simulink model "TruckBenchmark"  (R2023a)
settings: Solver=FixedStepAuto  StartTime=0.0  StopTime=sim_time  FixedStep=control.Ts  MaxStep=1  RelTol=1e-3  EnableMultiTasking=on
StartFcn:
  | tic
StopFcn:
  | simt=toc;
  | fprintf('Simulation time %.3f s\n',simt)
  | TruckBenchmark_Evaluation
values from neighbouring files (symbols this model uses):
  attack_duration = input('Enter the duration of each attack: ')    [RunMe.m]
  attack_freq = input('Enter the desired frequency of attack: ')    [RunMe.m]
  attack_time = input('Enter the time for attack: ')    [RunMe.m]
  attack_type = input('Select the type of Attack (1= Fuzzy, 2=spoofing, 3=Plateau, 4=Replay Attack, 5 = GAttack, 6= C-GAttack, 7= No Attack, 8 = Denial of Service):')    [RunMe.m]
  can_sample_time = 0.001    [runSim.m]
  clutch_pos = TruckBenchmark_Result.find('clutch_pos').Values    [TruckBenchmark_Evaluation.m]
  control =     [TruckBenchmark_Control.mat]
  cruise_profile = input('Select Cruise Profile (Step decrease = 1, Constant 80kph = 2): ')    [RunMe.m]
  curr_gear = TruckBenchmark_Result.find('curr_gear').Values    [TruckBenchmark_Evaluation.m]
  DoS = 0    [RunMe.m]
  gattack_data = interp1(original_time, data, desired_time, 'linear')    [RunMe.m]
  gattack_time = desired_time    [RunMe.m]
  k_slope = TruckBenchmark_Result.find('k_slope').Values    [TruckBenchmark_Evaluation.m]
  lambda = TruckBenchmark_Result.find('lambda').Values    [TruckBenchmark_Evaluation.m]
  model =     [TruckBenchmark_Data.mat]
  n_engine = TruckBenchmark_Result.find('n_engine').Values    [TruckBenchmark_Evaluation.m]
  road = scenario.road    [runSim.m]
  scenario =     [Sodertalje_Norrkoping_Scenario.mat]
  sim_time = input('Enter the total simulation time: ')    [RunMe.m]
  spoofed_value = input('Set the spoofing value:')    [RunMe.m]
  ts = struct('orig_30kph', ts_orig_30kph, 'gen_30kph', ts_gen_30kph, 'orig_40kph', ts_orig_40kph, 'gen_40kph', ts_gen_40kph, 'orig_50kph', ts_orig_50kph, 'gen_50kph', ts_gen_50kph, 'orig_60kph', ts_orig_60kph, 'gen_60kph', ts_gen_60kph,'orig_70kph', ts_orig_70kph, 'gen_70kph', ts_gen_70kph, 'orig_80kph', ts_orig_80kph, 'gen_80kph', ts_gen_80kph, 'orig_90kph', ts_orig_90kph, 'gen_90kph', ts_gen_90kph)    [data_to_mat.m]
  v_vehicle = 0    [RunMe.m]    (also in TruckBenchmark_Evaluation.m = TruckBenchmark_Result.find('v_vehicle').Values)
undefined symbols (not defined in the file or in its folder): canChannel, CCVS, DiscIntNeverNeededParam, dm_airInlet, EGF1, ESSI, ETC2, gcbh, IMT1, n_t, p_inletManifold, r_egr, VD, VDHR, x_distance
libraries: j1939protocollib x25, simulink x5, canlib x2, j1939tllib x2, canmsglib x1, vntj1939tllib x1, slpidlib x1
(part 3 of 4)

== system TruckBenchmark/Controller/CAN TX//RX/J1939 CAN Transport Layer3 ==
  CAN Configuration : S-Function  LoadFcn=set_param(gcb, 'BlockHandle', num2str(gcbh));  FunctionName=svntcanconfig  Parameters=BlockHandle, Device, ObjConstructor, BusSpeed, EnableBitParameters, SJW, TSEG1, TSEG2, NSamples, AckMode  SFunctionDeploymentMode=off  EnableBusSupport=off  mask(CAN Configuration){BlockHandle=865.0001, Device=MathWorks Virtual 1 (Channel 2), ObjConstructor=canChannel('MathWorks', 'Virtual 1', 2), BusSpeed=250000, EnableBitParameters=off, SJW=1, TSEG1=4, TSEG2=3, NSamples=1, AckMode=Normal}
      mask prompts: BlockHandle "Block handle"; Device "Device Name"; ObjConstructor "Object constructor"; BusSpeed "Bus speed:"; EnableBitParameters "Set bit parameters manually"; SJW "Synchronization jump width (SJW):"; TSEG1 "Time segment 1 (TSEG1)"; TSEG2 "Time segment 2 (TSEG2)"; NSamples "Number of samples:"; AckMode "Acknowledge mode:"
      mask help: Configure the properties for the specified CAN device.
      mask Help: eval('helpview(fullfile(docroot, ''toolbox'', ''vnt'', ''vnt.map''), ''vnt_canconfig_block'')');
      mask TypeOptions AckMode: Normal | Silent
  CAN Receive : S-Function  LoadFcn=set_param(gcb, 'BlockHandle', num2str(gcbh));  FunctionName=svntcanreceive  Parameters=BlockHandle, Device, ObjConstructor, EnableStandardIDsFilter, StandardIDs, EnableExtendedIDsFilter, ExtendedIDs, SampleTime, MsgsPerTimestep, StdIDsCombo, ExtIDsCombo, InternalFilterUpdateStatus, BusOutput  SFunctionDeploymentMode=off  EnableBusSupport=off  mask(CAN Receive){BlockHandle=866.0004, Device=MathWorks Virtual 1 (Channel 2), ObjConstructor=canChannel('MathWorks', 'Virtual 1', 2), EnableStandardIDsFilter=off, StandardIDs=0, EnableExtendedIDsFilter=off, ExtendedIDs=0, SampleTime=can_sample_time, MsgsPerTimestep=all, StdIDsCombo=Allow all, ExtIDsCombo=Allow all, InternalFilterUpdateStatus=on, BusOutput=off}
      mask prompts: BlockHandle "Block handle"; Device "Device Name"; ObjConstructor "Object constructor"; EnableStandardIDsFilter "Filter for accepted Standard ID range"; StandardIDs "Standard IDs"; EnableExtendedIDsFilter "Filter for accepted Extended ID range"; ExtendedIDs "Extended IDs"; SampleTime "Sample time:"; MsgsPerTimestep "Messages per timestep"; StdIDsCombo "Standard IDs Combo"; ExtIDsCombo "Extended IDs Combo"; InternalFilterUpdateStatus "Internal Filter update"; BusOutput "Output as bus"
      mask help: Receive CAN Messages using the specified CAN device.
      mask Help: eval('helpview(fullfile(docroot, ''toolbox'', ''vnt'', ''vnt.map''), ''vnt_canrec_block'')');
      mask TypeOptions MsgsPerTimestep: 1 | all
      mask TypeOptions StdIDsCombo: Allow all | Allow only | Block only
      mask TypeOptions ExtIDsCombo: Allow all | Allow only | Block only
  CAN Transmit Subsystem : Subsystem  TreatAsAtomicUnit=on
  Data Type Conversion : DataTypeConversion  Commented=on  SaturateOnIntegerOverflow=off  RndMeth=Floor
  J1939 Transport Layer Transmit : S-Function  FunctionName=slcantx  Parameters=TLID, TLTag, MaxNumMessages, SampleTime  SFunctionDeploymentMode=off  EnableBusSupport=off  mask(J1939 Transport Layer Transmit){TLID=Config2, MaxNumMessages=20, SampleTime=can_sample_time}
      mask prompts: TLID "Config ID:"; MaxNumMessages "Maximum number of messages:"; SampleTime "Sample time:"
      mask help:
      | Processes the queued J1939 messages and sends to the
      | protocol (CAN) transmit block for transmission.
      mask init:
      | [str, port] = j1939.internal.getTLDisplayString;
      | TLTag = j1939.internal.getTLParams;
      mask Help: uiwait(warndlg('Yet to be tagged'));
      mask Display:
      | disp(str);
      | port_label('output',port(1).id,port(1).label);
      | port_label('output',port(2).id,port(2).label);
  J1939 Transport Layer Receive Subsystem : Subsystem  TreatAsAtomicUnit=on
  To Workspace : ToWorkspace  Commented=on  VariableName=can_raw_data  SaveFormat=Timeseries  SampleTime=-1
      settings: Save2DSignal=2-D array (concatenate along first dimension)
  wires:
  J1939 Transport Layer Transmit/1 -> Data Type Conversion/1, CAN Transmit Subsystem/1(CAN Msg)
  J1939 Transport Layer Transmit/2 -> CAN Transmit Subsystem/2(N)
  CAN Receive/2 -> J1939 Transport Layer Receive Subsystem/1(In1)
  CAN Receive/1 -> J1939 Transport Layer Receive Subsystem/Trigger
  Data Type Conversion/1 -> To Workspace/1

== system TruckBenchmark/Vehicle Model/Chassi/Aerodynamic  resistance ==
  v [m/s] : Inport
  0.5*rho_air*A*C_d : Gain  Gain=0.5*rho*C_d*Area  SaturateOnIntegerOverflow=on  OutDataTypeStr=Inherit: Same as input  ParamDataTypeStr=Inherit: Same as input
  v^2 : Math  Operator=square  SignedPower=on
  F_a : Outport  VectorParamsAs1DForOutWhenUnconnected=off
  wires:
  v [m/s]/1 -> v^2/1
  v^2/1 -> 0.5*rho_air*A*C_d/1
  0.5*rho_air*A*C_d/1 -> F_a/1  "F_a"

== system TruckBenchmark/Vehicle Model/Chassi/Gravitational force ==
  alpha [rad] : Inport
  Trigonometric Function : Trigonometry
  m g : Constant  Value=m*g
  mult2 : Product  SaturateOnIntegerOverflow=on  OutDataTypeStr=Inherit: Same as first input
  F_g : Outport  VectorParamsAs1DForOutWhenUnconnected=off
  wires:
  alpha [rad]/1 -> Trigonometric Function/1
  m g/1 -> mult2/2
  mult2/1 -> F_g/1  "F_g"
  Trigonometric Function/1 -> mult2/1

== system TruckBenchmark/Vehicle Model/Chassi/Rolling resistance ==
  v [m/s] : Inport
  alpha [rad] : Inport  Port=2
  Math Function : Math  Operator=square  SignedPower=on
  Sum1 : Sum  SaturateOnIntegerOverflow=on
  Trigonometric Function : Trigonometry  Operator=cos
  c_r0 : Constant  Value=c_r0
  c_r1 : Constant  Value=c_r1
  const : Constant  Value=3.6
  m g : Constant  Value=m*g
  mult{,1..3} (4 alike) : Product  SaturateOnIntegerOverflow=on  OutDataTypeStr=Inherit: Same as first input
  F_r : Outport  VectorParamsAs1DForOutWhenUnconnected=off
  wires:
  v [m/s]/1 -> mult3/1
  Sum1/1 -> mult1/1
  mult1/1 -> F_r/1  "F_r"
  c_r0/1 -> Sum1/2
  mult/1 -> Sum1/1
  c_r1/1 -> mult/2
  m g/1 -> mult2/2
  alpha [rad]/1 -> Trigonometric Function/1
  mult2/1 -> mult1/2
  Trigonometric Function/1 -> mult2/1
  const/1 -> mult3/2
  mult3/1 -> Math Function/1  "v [km/h]"
  Math Function/1 -> mult/1

== system TruckBenchmark/Vehicle Model/Clutch and Transmission/Clutch Transfer ==
  Tq_c_max : Inport
  Clutch Locked : Inport  Port=2
  Insignals : Inport  Port=3
  Abs : Abs
  Abs1 : Abs
  Calc Mc : Fcn  Expr=(u(1)*u(4)/(u(5)^2) + u(2)*u(3)/u(5)) / (u(2) + u(4)/(u(5)^2))
  Logical Operator : Logic  AllPortsSameDT=off  OutDataTypeStr=boolean
  Relational Operator : RelationalOperator  Operator=<  OutDataTypeStr=boolean  InputSameDT=off
  Switch : Switch  Threshold=0.5
  M_c : Outport  VectorParamsAs1DForOutWhenUnconnected=off
  wires:
  Switch/1 -> M_c/1
  Calc Mc/1 -> Abs/1, Switch/1
  Insignals/1 -> Calc Mc/1
  Tq_c_max/1 -> Abs1/1, Switch/3
  Logical Operator/1 -> Switch/2
  Clutch Locked/1 -> Logical Operator/1
  Abs/1 -> Relational Operator/1
  Abs1/1 -> Relational Operator/2
  Relational Operator/1 -> Logical Operator/2

== system TruckBenchmark/Vehicle Model/Clutch and Transmission/Engine Dynamics ==
  Tq_c : Inport
  Tq_e : Inport  Port=2
  J_e : Inport  Port=3
  Integrator1 : Integrator  InitialCondition=600*pi/30  LimitOutput=on  LowerSaturationLimit=450*pi/30
  Sum2 : Sum  Inputs=-+|  InputSameDT=on  SaturateOnIntegerOverflow=on  OutDataTypeStr=Inherit: Same as first input
  w dot4 : Product  Inputs=*/  InputSameDT=on  SaturateOnIntegerOverflow=on  OutDataTypeStr=Inherit: Same as first input
  w_e : Outport  VectorParamsAs1DForOutWhenUnconnected=off
  wires:
  w dot4/1 -> Integrator1/1
  Sum2/1 -> w dot4/1
  J_e/1 -> w dot4/2
  Integrator1/1 -> w_e/1
  Tq_c/1 -> Sum2/1
  Tq_e/1 -> Sum2/2

== system TruckBenchmark/Vehicle Model/Clutch and Transmission/Speed Difference Clutch Limits ==
  Clutch [0...1] : Inport
  w_e : Inport  Port=2
  w_wheel : Inport  Port=3
  Gear ratio : Inport  Port=4
  Abs : Abs
  Compare To Zero : simulink/Logic and Bit Operations/Compare To Zero  relop=>  OutDataTypeStr=uint8
  Data Type Conversion : DataTypeConversion  SaturateOnIntegerOverflow=off  RndMeth=Floor
  Maximum Transmissable Clutch Torque : Gain  Gain=model.clutch.M_max  SaturateOnIntegerOverflow=on  OutDataTypeStr=Inherit: Same as input  ParamDataTypeStr=Inherit: Same as input
  Mux1 : Mux  Inputs=3
  Product : Product  Inputs=3  InputSameDT=on  SaturateOnIntegerOverflow=on  OutDataTypeStr=Inherit: Same as first input
  Product1 : Product  InputSameDT=on  SaturateOnIntegerOverflow=on  OutDataTypeStr=Inherit: Same as first input
  Relay1 : Relay  OnSwitchValue=1  OffSwitchValue=1e-1  OnOutputValue=0  OffOutputValue=1
  Relay2 : Relay  OnSwitchValue=1e-1  OffSwitchValue=-1e-1  OffOutputValue=-1
  Sum : Sum  Inputs=|+-  InputSameDT=on  SaturateOnIntegerOverflow=on  OutDataTypeStr=Inherit: Same as first input
  To Workspace : ToWorkspace  VariableName=C  SaveFormat=Structure With Time  SampleTime=-1
  Clutch Locked : Outport  VectorParamsAs1DForOutWhenUnconnected=off
  M_c_max : Outport  Port=2  VectorParamsAs1DForOutWhenUnconnected=off
  wires:
  Relay2/1 -> Product/3, Mux1/2
  Abs/1 -> Relay1/1
  Sum/1 -> Relay2/1, Abs/1
  Clutch [0...1]/1 -> Maximum Transmissable Clutch Torque/1
  w_e/1 -> Sum/1
  Gear ratio/1 -> Compare To Zero/1, Product1/2
  w_wheel/1 -> Product1/1
  Maximum Transmissable Clutch Torque/1 -> Product/1
  Relay1/1 -> Clutch Locked/1, Mux1/3
  Mux1/1 -> To Workspace/1
  Product/1 -> Mux1/1, M_c_max/1
  Product1/1 -> Sum/2
  Compare To Zero/1 -> Data Type Conversion/1
  Data Type Conversion/1 -> Product/2

== system TruckBenchmark/Vehicle Model/Clutch and Transmission/Vehicle Dynamics ==
  Tq_c : Inport
  Tq_veh : Inport  Port=2
  J_v : Inport  Port=3
  Gear ratio : Inport  Port=4
  Integrator : Integrator  LimitOutput=on  LowerSaturationLimit=0
  Sum1 : Sum  Inputs=|+-  InputSameDT=on  SaturateOnIntegerOverflow=on  OutDataTypeStr=Inherit: Same as first input
  w dot3 : Product  Inputs=**  InputSameDT=on  SaturateOnIntegerOverflow=on  OutDataTypeStr=Inherit: Same as first input
  w dot5 : Product  Inputs=*/  InputSameDT=on  SaturateOnIntegerOverflow=on  OutDataTypeStr=Inherit: Same as first input
  w_wheel : Outport  VectorParamsAs1DForOutWhenUnconnected=off
  wires:
  Gear ratio/1 -> w dot3/2
  J_v/1 -> w dot5/2
  Tq_c/1 -> w dot3/1
  Tq_veh/1 -> Sum1/2
  w dot3/1 -> Sum1/1
  Sum1/1 -> w dot5/1
  w dot5/1 -> Integrator/1
  Integrator/1 -> w_wheel/1

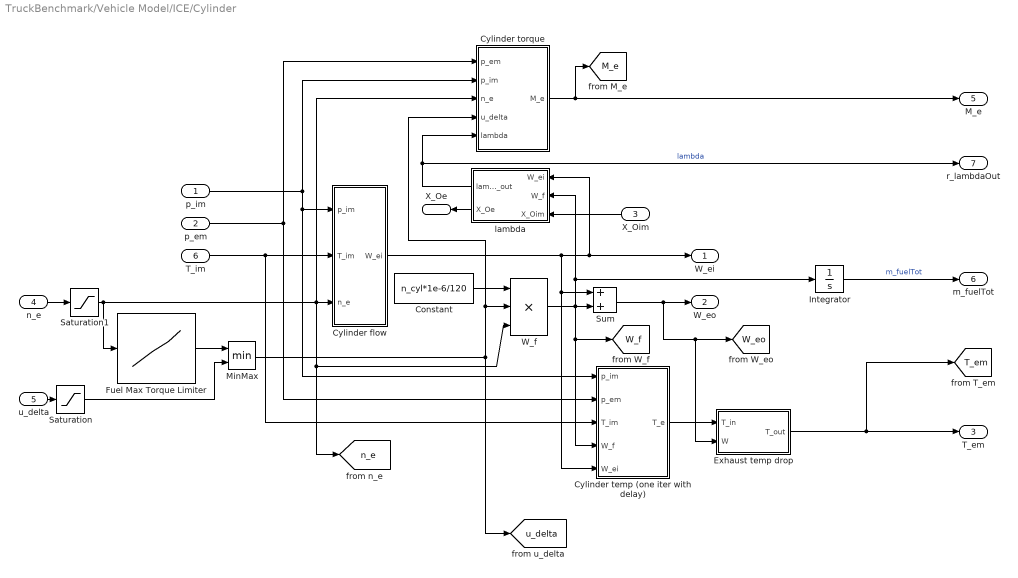
== system TruckBenchmark/Vehicle Model/ICE/Cylinder ==
  p_im : Inport
  p_em : Inport  Port=2
  X_Oim : Inport  Port=3
  n_e : Inport  Port=4
  u_delta : Inport  Port=5
  T_im : Inport  Port=6
  Constant : Constant  Value=n_cyl*1e-6/120
  Cylinder flow : Subsystem  mask{c_volVec=model.engine.c_volVec}
  Cylinder temp (one iter with delay) : Subsystem  mask{x_cv=model.engine.x_cv, eta_sc=model.engine.eta_sc, x_r_Init=model.engine.x_r_Init, T_1_Init=model.engine.T_1_Init}
  Cylinder torque : Subsystem  mask{c_fricVec=model.engine.c_fricVec, eta_igch=model.engine.eta_igch, gamma_c=model.engine.gamma_c}
  Exhaust temp drop : Subsystem  mask{h_tot=model.engine.h_tot, n_pipe=model.engine.n_pipe, l_pipe=model.engine.l_pipe, d_pipe=model.engine.d_pipe, T_w=model.engine.T_w}
  Fuel Max Torque Limiter : Lookup_n-D  NumberOfTableDimensions=1  BreakpointsForDimension1=limit_n_e  Table=limit_m_f  RndMeth=Simplest
  Integrator : Integrator
  MinMax : MinMax  Inputs=2
  Saturation : Saturate  UpperLimit=340  LowerLimit=0
  Saturation1 : Saturate  UpperLimit=2000  LowerLimit=400
  Sum : Sum  SaturateOnIntegerOverflow=on
  W_f : Product  Inputs=3  SaturateOnIntegerOverflow=on  OutDataTypeStr=Inherit: Same as first input
  lambda : Subsystem
  W_ei : Outport  VectorParamsAs1DForOutWhenUnconnected=off
  W_eo : Outport  Port=2  VectorParamsAs1DForOutWhenUnconnected=off
  T_em : Outport  Port=3  VectorParamsAs1DForOutWhenUnconnected=off
  X_Oe : Outport  Port=4  VectorParamsAs1DForOutWhenUnconnected=off
  M_e : Outport  Port=5  VectorParamsAs1DForOutWhenUnconnected=off
  m_fuelTot : Outport  Port=6  VectorParamsAs1DForOutWhenUnconnected=off
  r_lambdaOut : Outport  Port=7  VectorParamsAs1DForOutWhenUnconnected=off
  tag scope: M_e=global, T_em=global, W_eo=global, W_f=global, n_e=global, u_delta=global
  wires:
  lambda/2(X_Oe) -> X_Oe/1
  n_e/1 -> Saturation1/1
  X_Oim/1 -> lambda/3(X_Oim)
  lambda/1(lambda_out) -> r_lambdaOut/1, Cylinder torque/5(lambda)  "lambda"
  Cylinder temp (one iter with delay)/1(T_e) -> Exhaust temp drop/1(T_in)
  Cylinder torque/1(M_e) -> [M_e], M_e/1
  u_delta/1 -> Saturation/1
  Constant/1 -> W_f/1
  W_f/1 -> Integrator/1, lambda/2(W_f), [W_f], Cylinder temp (one iter with delay)/4(W_f), Sum/2
  Sum/1 -> Exhaust temp drop/2(W), [W_eo], W_eo/1
  Cylinder flow/1(W_ei) -> lambda/1(W_ei), W_ei/1, Cylinder temp (one iter with delay)/5(W_ei), Sum/1
  T_im/1 -> Cylinder temp (one iter with delay)/3(T_im), Cylinder flow/2(T_im)
  p_em/1 -> Cylinder temp (one iter with delay)/2(p_em), Cylinder torque/1(p_em)
  p_im/1 -> Cylinder temp (one iter with delay)/1(p_im), Cylinder flow/1(p_im), Cylinder torque/2(p_im)
  Exhaust temp drop/1(T_out) -> [T_em], T_em/1
  Saturation1/1 -> Fuel Max Torque Limiter/1, Cylinder flow/3(n_e), [n_e], W_f/3, Cylinder torque/3(n_e)
  Integrator/1 -> m_fuelTot/1  "m_fuelTot"
  Saturation/1 -> MinMax/2
  Fuel Max Torque Limiter/1 -> MinMax/1
  MinMax/1 -> Cylinder torque/4(u_delta), W_f/2, [u_delta]

== system TruckBenchmark/Vehicle Model/ICE/EGR-system ==
  p_im : Inport
  T_em : Inport  Port=2
  p_em : Inport  Port=3
  u_egr : Inport  Port=4
  Constant : Constant  Value=model.engine.with_egr_act_model
  EGR act : Subsystem
  Fcn W_egr : Fcn  Expr=A_egrmax*u[1]*u[3]*u[2]/sqrt(u[4]*R_e)
  Mux : Mux
  PI_egr : Product  Inputs=*/  SaturateOnIntegerOverflow=on  OutDataTypeStr=Inherit: Same as first input
  PSI_egr : Subsystem
  Saturation : Saturate  UpperLimit=100  LowerLimit=0
  Switch : Switch  Threshold=0.5  InputSameDT=off
  f_egr : Subsystem
  W_egr : Outport  VectorParamsAs1DForOutWhenUnconnected=off
  tag scope: W_egr=global, u_egr=global, u_egract=global
  wires:
  Constant/1 -> Switch/2
  EGR act/1(Out) -> Switch/1
  Switch/1 -> [u_egract], f_egr/1(u_egr)
  u_egr/1 -> Saturation/1
  Fcn W_egr/1 -> [W_egr], W_egr/1
  T_em/1 -> Mux/4
  PSI_egr/1(PSI_egr) -> Mux/2
  f_egr/1(f_egr) -> Mux/1
  Mux/1 -> Fcn W_egr/1
  PI_egr/1 -> PSI_egr/1(PI_egr)
  p_em/1 -> Mux/3, PI_egr/2
  p_im/1 -> PI_egr/1
  Saturation/1 -> EGR act/1(In), Switch/3, [u_egr]

== system TruckBenchmark/Vehicle Model/ICE/Exhaust Manifold ==
  W_eo : Inport
  W_t : Inport  Port=2
  W_egr : Inport  Port=3
  T_em : Inport  Port=4
  X_Oe : Inport  Port=5
  Fcn : Fcn  Expr=R_e*u[1]*u[2]/V_em
  Integrator p_em : Integrator  InitialCondition=p_em_Init  LimitOutput=on  UpperSaturationLimit=20*p_amb  LowerSaturationLimit=0.5*p_amb
  Mux : Mux  Inputs=2
  Subsystem : Subsystem
  Sum : Sum  Inputs=+--  SaturateOnIntegerOverflow=on
  p_em : Outport  VectorParamsAs1DForOutWhenUnconnected=off
  X_Oem : Outport  Port=2  VectorParamsAs1DForOutWhenUnconnected=off
  tag scope: X_Oem=global, p_em=global
  wires:
  Subsystem/1(X_Oem) -> [X_Oem], X_Oem/1
  X_Oe/1 -> Subsystem/4(X_Oe)
  Integrator p_em/1 -> Subsystem/1(p_em), [p_em], p_em/1
  W_eo/1 -> Subsystem/3(W_eo), Sum/1
  W_t/1 -> Sum/2
  W_egr/1 -> Sum/3
  Sum/1 -> Mux/1
  T_em/1 -> Subsystem/2(T_em), Mux/2
  Mux/1 -> Fcn/1
  Fcn/1 -> Integrator p_em/1

== system TruckBenchmark/Vehicle Model/ICE/Intake Manifold ==
  W_c : Inport
  W_egr : Inport  Port=2
  W_ei : Inport  Port=3
  T_im : Inport  Port=4
  X_Oem : Inport  Port=5
  Constant1 : Constant  Value=0.9
  Fcn : Fcn  Expr=R_a*u[1]*u[2]/V_im
  Integrator p_im : Integrator  InitialCondition=p_im_Init  LimitOutput=on  UpperSaturationLimit=10*p_amb  LowerSaturationLimit=0.5*p_amb
  MinMax1 : MinMax  Inputs=2  InputSameDT=on  SaturateOnIntegerOverflow=on
  Mux : Mux  Inputs=2
  Product : Product  Inputs=*/  SaturateOnIntegerOverflow=on  OutDataTypeStr=Inherit: Same as first input
  Subsystem X_Oim : Subsystem
  Sum : Sum  Inputs=+-  SaturateOnIntegerOverflow=on
  Sum1 : Sum  SaturateOnIntegerOverflow=on
  p_im : Outport  VectorParamsAs1DForOutWhenUnconnected=off
  X_Oim : Outport  Port=2  VectorParamsAs1DForOutWhenUnconnected=off
  r_egr : Outport  Port=3  VectorParamsAs1DForOutWhenUnconnected=off
  tag scope: X_Oim=global, p_im=global, x_egr=global
  wires:
  Subsystem X_Oim/1(X_Oim) -> [X_Oim], X_Oim/1
  X_Oem/1 -> Subsystem X_Oim/5(X_Oem)
  Product/1 -> r_egr/1, MinMax1/1  "r_egr"
  Constant1/1 -> MinMax1/2
  W_egr/1 -> Subsystem X_Oim/3(W_egr), Product/1, Sum1/2
  W_c/1 -> Subsystem X_Oim/4(W_c), Sum1/1
  Sum1/1 -> Product/2, Sum/1
  Fcn/1 -> Integrator p_im/1
  Mux/1 -> Fcn/1
  T_im/1 -> Subsystem X_Oim/2(T_im), Mux/2
  Sum/1 -> Mux/1
  W_ei/1 -> Sum/2
  Integrator p_im/1 -> Subsystem X_Oim/1(p_im), [p_im], p_im/1
  MinMax1/1 -> [x_egr]

== system TruckBenchmark/Vehicle Model/ICE/Turbo ==
  p_im : Inport
  p_em : Inport  Port=2
  T_em : Inport  Port=3
  u_vgt : Inport  Port=4
  Compressor : Subsystem  mask{c_pi=model.engine.c_pi, pi_copt=model.engine.pi_copt, w_copt=model.engine.w_copt, eta_cmax=model.engine.eta_cmax, Q_c=model.engine.Q_c, c_wphiVec=model.engine.c_wphiVec, c_wpsiVec=model.engine.c_wpsiVec, c_phi2=model.engine.c_phi2, c_psi2=model.engine.c_psi2, R_c=model.engine.R_c}
  Turbine : Subsystem  mask{c_vgt2=model.engine.c_vgt2, c_vgt1=model.engine.c_vgt1, c_f2=model.engine.c_f2, c_f1=model.engine.c_f1, K_t=model.engine.K_t, uInit_vgt=model.engine.uInit_vgt, tau_vgt=model.engine.tau_vgt, c_mlin=model.engine.c_mlin, w_tlin=model.engine.w_tlin, c_mVec=model.engine.c_mVec, BSR_opt=model.engine.BSR_opt, eta_tmmax=model.engine.eta_tmmax, R_t=model.engine.R_t, A_vgtmax=model.engine.A_vgtmax}
  Turbo inertia : Subsystem  mask{omega_t_Init=model.engine.omega_t_Init, J_t=model.engine.J_t}
  amb pres : Constant  Value=p_amb
  amb temp : Constant  Value=T_amb
  "rad/s -> RPM" : Gain  Gain=30/pi  SaturateOnIntegerOverflow=on  OutDataTypeStr=Inherit: Same as input  ParamDataTypeStr=Inherit: Same as input
  W_c : Outport  VectorParamsAs1DForOutWhenUnconnected=off
  T_c : Outport  Port=2  VectorParamsAs1DForOutWhenUnconnected=off
  W_t : Outport  Port=3  VectorParamsAs1DForOutWhenUnconnected=off
  n_t : Outport  Port=4  VectorParamsAs1DForOutWhenUnconnected=off
  wires:
  u_vgt/1 -> Turbine/5(u_vgt)
  T_em/1 -> Turbine/1(T_em)
  p_em/1 -> Turbine/2(p_em)
  Turbine/1(W_t) -> W_t/1
  Compressor/2(T_c) -> T_c/1
  Compressor/1(W_c) -> W_c/1
  Compressor/3(P_c) -> Turbo inertia/2(P_c)
  Turbine/2(P_t*eta_m) -> Turbo inertia/1(P_t*eta_m)
  Turbo inertia/1(omega_t) -> Turbine/4(omega_t), "rad/s -> RPM"/1, Compressor/4(omega_t)
  p_im/1 -> Compressor/3(p_c)
  amb pres/1 -> Turbine/3(p_es), Compressor/2(p_bc)
  amb temp/1 -> Compressor/1(T_bc)
  "rad/s -> RPM"/1 -> n_t/1  "n_t"

== system TruckBenchmark/Controller/CAN TX//RX/ Periodic Trigger1/Timer ==
  Reset : Inport
  Constant : Constant  Value=eps
  Gain : Gain  Gain=1e3
  Logical Operator : Logic  Operator=NOT  AllPortsSameDT=off  OutDataTypeStr=boolean
  MATLAB Function : MATLAB Function  TreatAsAtomicUnit=on
  Sum : Sum  Inputs=-+
  Sum1 : Sum  Inputs=|++
  Switch : Switch  Criteria=u2 > Threshold  ZeroCross=off  SaturateOnIntegerOverflow=off  InputSameDT=off
  Unit Delay : UnitDelay  SampleTime=-1  HasFrameUpgradeWarning=on
  Unit Delay1 : UnitDelay  SampleTime=-1  HasFrameUpgradeWarning=on
  Timer Value (ms) : Outport  VectorParamsAs1DForOutWhenUnconnected=off
  wires:
  Gain/1 -> Timer Value (ms)/1
  Constant/1 -> Sum1/2
  Sum1/1 -> Gain/1
  Sum/1 -> Sum1/1
  Logical Operator/1 -> Switch/2
  MATLAB Function/1(y) -> Sum/2, Unit Delay1/1
  Unit Delay1/1 -> Switch/3
  Switch/1 -> Unit Delay/1, Sum/1
  Unit Delay/1 -> Switch/1
  Reset/1 -> Logical Operator/1

== system TruckBenchmark/Controller/CAN TX//RX/Attack Block/C-GAttack Block ==
  Speed : Inport
  If : If  IfExpression=u1 <= 30  ElseIfExpressions=u1 >= 31 & u1<=40,u1 >= 41 & u1<=50,u1 >= 51 & u1<=60,u1 >= 61 & u1<=70,u1 >= 71 & u1<=80,u1 >= 81 & u1<=90  ShowElse=off
  If Action Subsystem : Subsystem  TreatAsAtomicUnit=on
  If Action Subsystem1 : Subsystem  TreatAsAtomicUnit=on
  If Action Subsystem2 : Subsystem  TreatAsAtomicUnit=on
  If Action Subsystem3 : Subsystem  TreatAsAtomicUnit=on
  If Action Subsystem4 : Subsystem  TreatAsAtomicUnit=on
  If Action Subsystem5 : Subsystem  TreatAsAtomicUnit=on
  If Action Subsystem6 : Subsystem  TreatAsAtomicUnit=on
  Merge : Merge  Inputs=7
  attack_data : Outport
  wires:
  If/5 -> If Action Subsystem4/Action
  If/4 -> If Action Subsystem3/Action
  If Action Subsystem1/1(AttachSpd_40) -> Merge/2
  If Action Subsystem3/1(AttachSpd_60) -> Merge/4
  If Action Subsystem/1(AttachSpd_30) -> Merge/1
  If Action Subsystem2/1(AttachSpd_50) -> Merge/3
  If/1 -> If Action Subsystem/Action
  If Action Subsystem4/1(AttachSpd_70) -> Merge/5
  If Action Subsystem6/1(AttachSpd_80) -> Merge/6
  If Action Subsystem5/1(AttackSpd_90) -> Merge/7
  If/6 -> If Action Subsystem6/Action
  Speed/1 -> If/1
  Merge/1 -> attack_data/1
  If/2 -> If Action Subsystem1/Action
  If/3 -> If Action Subsystem2/Action
  If/7 -> If Action Subsystem5/Action

== system TruckBenchmark/Controller/CAN TX//RX/Attack Block/If Action Subsystem ==
  1-D Lookup Table : Lookup_n-D  NumberOfTableDimensions=1  BreakpointsForDimension1=gattack_time  Table=gattack_data  InternalRulePriority=Speed  RndMeth=Simplest
  Clock : Clock
  GAttack : Outport
  wires:
  Clock/1 -> 1-D Lookup Table/1
  1-D Lookup Table/1 -> GAttack/1

== system TruckBenchmark/Controller/CAN TX//RX/Attack Block/Plateau Attack ==
  v_vehicle : Inport
  Memory : Memory
  Pulse Generator : DiscretePulseGenerator  PulseType=Time based  Period=100  PulseWidth=50  PhaseDelay=attack_time
  Step : Step  Commented=on  Time=attack_time  SampleTime=0
  Switch : Switch  Criteria=u2 > Threshold  SaturateOnIntegerOverflow=off  InputSameDT=off
  Out1 : Outport
  wires:
  Memory/1 -> Switch/1
  Switch/1 -> Memory/1, Out1/1
  v_vehicle/1 -> Switch/3
  Step/1 -> ?
  Pulse Generator/1 -> Switch/2

== system TruckBenchmark/Controller/CAN TX//RX/J1939 CAN Transport Layer1/CAN Transmit Subsystem ==
  CAN Msg : Inport
  N : Inport  Port=2
  CAN Transmit : S-Function  LoadFcn=set_param(gcb, 'BlockHandle', num2str(gcbh));  FunctionName=svntcantransmit  Parameters=BlockHandle, Device, ObjConstructor,EnablePeriodicTransmit,MessagePeriod,EnableEventTransmit  SFunctionDeploymentMode=off  EnableBusSupport=off  mask(CAN Transmit){BlockHandle=833.0001, Device=MathWorks Virtual 1 (Channel 1), ObjConstructor=canChannel('MathWorks', 'Virtual 1', 1), EnableEventTransmit=off, EnablePeriodicTransmit=off, MessagePeriod=1.000}
      mask prompts: BlockHandle "Block handle"; Device "Device Name"; ObjConstructor "Object Constructor:"; EnableEventTransmit "On data change"; EnablePeriodicTransmit "Transmit messages periodically"; MessagePeriod "Message period (in seconds):"
      mask help: Transmit CAN Messages using the specified CAN device.
      mask Help: eval('helpview(fullfile(docroot, ''toolbox'', ''vnt'', ''vnt.map''), ''vnt_cantran_block'')');
  For Iterator : ForIterator  IterationSource=external
  Index Vector : MultiPortSwitch  Inputs=1  SaturateOnIntegerOverflow=off  InputSameDT=off
  wires:
  N/1 -> For Iterator/1
  For Iterator/1 -> Index Vector/1
  CAN Msg/1 -> Index Vector/2
  Index Vector/1 -> CAN Transmit/1

== system TruckBenchmark/Controller/CAN TX//RX/J1939 CAN Transport Layer1/J1939 Transport Layer Receive Subsystem ==
  In1 : Inport
  function : TriggerPort  TriggerType=function-call  VariantControl=Variant
  Constant : Constant
  J1939 Transport Layer Receive : j1939tllib/J1939 Transport Layer Receive  TLID=Config1  MaxNumMessages=1  SampleTime=-1
  wires:
  Constant/1 -> J1939 Transport Layer Receive/2
  In1/1 -> J1939 Transport Layer Receive/1

== system TruckBenchmark/Controller/CAN TX//RX/J1939 CAN Transport Layer3/CAN Transmit Subsystem ==
  CAN Msg : Inport
  N : Inport  Port=2
  CAN Transmit : S-Function  LoadFcn=set_param(gcb, 'BlockHandle', num2str(gcbh));  FunctionName=svntcantransmit  Parameters=BlockHandle, Device, ObjConstructor,EnablePeriodicTransmit,MessagePeriod,EnableEventTransmit  SFunctionDeploymentMode=off  EnableBusSupport=off  mask(CAN Transmit){BlockHandle=873.0001, Device=MathWorks Virtual 1 (Channel 2), ObjConstructor=canChannel('MathWorks', 'Virtual 1', 2), EnableEventTransmit=off, EnablePeriodicTransmit=off, MessagePeriod=1.000}
      mask prompts: BlockHandle "Block handle"; Device "Device Name"; ObjConstructor "Object Constructor:"; EnableEventTransmit "On data change"; EnablePeriodicTransmit "Transmit messages periodically"; MessagePeriod "Message period (in seconds):"
      mask help: Transmit CAN Messages using the specified CAN device.
      mask Help: eval('helpview(fullfile(docroot, ''toolbox'', ''vnt'', ''vnt.map''), ''vnt_cantran_block'')');
  For Iterator : ForIterator  IterationSource=external
  Index Vector : MultiPortSwitch  Inputs=1  SaturateOnIntegerOverflow=off  InputSameDT=off
  wires:
  N/1 -> For Iterator/1
  For Iterator/1 -> Index Vector/1
  CAN Msg/1 -> Index Vector/2
  Index Vector/1 -> CAN Transmit/1

== system TruckBenchmark/Controller/CAN TX//RX/J1939 CAN Transport Layer3/J1939 Transport Layer Receive Subsystem ==
  In1 : Inport
  function : TriggerPort  TriggerType=function-call  VariantControl=Variant
  Constant : Constant
  J1939 Transport Layer Receive : j1939tllib/J1939 Transport Layer Receive  TLID=Config2  MaxNumMessages=1  SampleTime=-1
  wires:
  Constant/1 -> J1939 Transport Layer Receive/2
  In1/1 -> J1939 Transport Layer Receive/1

== system TruckBenchmark/Vehicle Model/ICE/Cylinder/Cylinder flow ==
  p_im : Inport
  T_im : Inport  Port=2
  n_e : Inport  Port=3
  Constant : Constant  Value=V_d/(R_a*60*2)
  Mux : Mux  Inputs=2
  Product W_ei : Product  Inputs=***/*  SaturateOnIntegerOverflow=on  OutDataTypeStr=Inherit: Same as first input
  n_vol : Fcn  Expr=c_volVec(1)*sqrt(u[1])+c_volVec(2)*sqrt(u[2])+c_volVec(3)
  W_ei : Outport  VectorParamsAs1DForOutWhenUnconnected=off
  tag scope: W_ei=global
  wires:
  Mux/1 -> n_vol/1
  Product W_ei/1 -> [W_ei], W_ei/1
  Constant/1 -> Product W_ei/5
  T_im/1 -> Product W_ei/4
  n_e/1 -> Mux/2, Product W_ei/3
  n_vol/1 -> Product W_ei/1
  p_im/1 -> Mux/1, Product W_ei/2

== system TruckBenchmark/Vehicle Model/ICE/Cylinder/Cylinder temp (one iter with delay) ==
  p_im : Inport
  p_em : Inport  Port=2
  T_im : Inport  Port=3
  W_f : Inport  Port=4
  W_ei : Inport  Port=5
  Constant : Constant  Value=1500
  MinMax : MinMax  Inputs=2  InputSameDT=on  SaturateOnIntegerOverflow=on
  Mux : Mux  Inputs=3
  Mux3 : Mux  Inputs=3
  PI_e : Product  Inputs=*/  SaturateOnIntegerOverflow=on  OutDataTypeStr=Inherit: Same as first input
  Saturation : Saturate  UpperLimit=1  LowerLimit=0
  Saturation1 : Saturate  UpperLimit=inf  LowerLimit=273
  Sub T_e : Subsystem
  T1 : Fcn  Expr=u[3]*u[1]+(1-u[3])*u[2]
  T_1Old : Memory  InitialCondition=T_1_Init  InheritSampleTime=on
  q_in : Fcn  Expr=u[1]*q_HV*(1-u[3])/(u[1]+u[2])
  x_p : Subsystem
  x_r : Subsystem
  x_rOld : Memory  InitialCondition=x_r_Init  InheritSampleTime=on
  T_e : Outport  VectorParamsAs1DForOutWhenUnconnected=off
  tag scope: T_1=global, T_e=global, x_r=global
  wires:
  Saturation1/1 -> T_1Old/1
  Saturation/1 -> x_rOld/1, Mux3/3
  Constant/1 -> MinMax/1
  Sub T_e/1(T_e) -> MinMax/2
  MinMax/1 -> [T_e], Mux3/1, T_e/1
  x_rOld/1 -> Mux/3, [x_r]
  x_r/1(x_r) -> Saturation/1
  T_1Old/1 -> [T_1], x_r/2(T1), x_p/2(T1), Sub T_e/3(T1)
  T1/1 -> Saturation1/1
  T_im/1 -> Mux3/2
  Mux3/1 -> T1/1
  x_p/1(x_p) -> x_r/1(x_p), Sub T_e/4(x_p)
  PI_e/1 -> x_r/4(PI_e), Sub T_e/1(PI_e)
  q_in/1 -> Sub T_e/2(q_in), x_p/1(q_in), x_r/3(q_in)
  W_ei/1 -> Mux/2
  W_f/1 -> Mux/1
  Mux/1 -> q_in/1
  p_em/1 -> PI_e/1
  p_im/1 -> PI_e/2

== system TruckBenchmark/Vehicle Model/ICE/Cylinder/Cylinder torque ==
  p_em : Inport
  p_im : Inport  Port=2
  n_e : Inport  Port=3
  u_delta : Inport  Port=4
  lambda : Inport  Port=5
  Constant : Constant
  Constant1 : Constant  Value=q_HV*1e-6*n_cyl
  Constant2 : Constant  Value=1-1/(r_c^(gamma_c-1))
  FMEP [bar] : Polyval  Coefs=c_fricVec
  Gain M_e : Gain  Gain=1/(4*pi)  SaturateOnIntegerOverflow=on  OutDataTypeStr=Inherit: Same as input  ParamDataTypeStr=Inherit: Same as input
  MinMax : MinMax  Inputs=2  InputSameDT=on  SaturateOnIntegerOverflow=on
  Sum : Sum  Inputs=-+  SaturateOnIntegerOverflow=on
  Sum1 : Sum  Inputs=+--  SaturateOnIntegerOverflow=on
  W_fric : Gain  Gain=V_d*1e5  SaturateOnIntegerOverflow=on  OutDataTypeStr=Inherit: Same as input  ParamDataTypeStr=Inherit: Same as input
  W_ig : Product  Inputs=4  SaturateOnIntegerOverflow=on  OutDataTypeStr=Inherit: Same as first input
  W_p : Gain  Gain=V_d  SaturateOnIntegerOverflow=on  OutDataTypeStr=Inherit: Same as input  ParamDataTypeStr=Inherit: Same as input
  gain : Gain  Gain=eta_igch  SaturateOnIntegerOverflow=on  OutDataTypeStr=Inherit: Same as input  ParamDataTypeStr=Inherit: Same as input
  n_eratio : Gain  Gain=1/1000  SaturateOnIntegerOverflow=on  OutDataTypeStr=Inherit: Same as input  ParamDataTypeStr=Inherit: Same as input
  M_e : Outport  VectorParamsAs1DForOutWhenUnconnected=off
  wires:
  Gain M_e/1 -> M_e/1  "M_e"
  Constant1/1 -> W_ig/4
  u_delta/1 -> W_ig/3
  Constant2/1 -> W_ig/2
  Sum1/1 -> Gain M_e/1
  W_fric/1 -> Sum1/3
  W_p/1 -> Sum1/2
  W_ig/1 -> Sum1/1
  FMEP [bar]/1 -> W_fric/1
  n_eratio/1 -> FMEP [bar]/1
  n_e/1 -> n_eratio/1
  gain/1 -> W_ig/1
  MinMax/1 -> gain/1
  Constant/1 -> MinMax/2
  lambda/1 -> MinMax/1
  Sum/1 -> W_p/1
  p_em/1 -> Sum/2
  p_im/1 -> Sum/1

== system TruckBenchmark/Vehicle Model/ICE/Cylinder/Exhaust temp drop ==
  T_in : Inport
  W : Inport  Port=2
  Fcn T_out : Fcn  Expr=T_w+(u[1]-T_w)*exp(-1*h_tot*pi*d_pipe*l_pipe*n_pipe/(u[2]*c_pe))
  Mux : Mux  Inputs=2
  T_out : Outport  VectorParamsAs1DForOutWhenUnconnected=off
  wires:
  Fcn T_out/1 -> T_out/1
  Mux/1 -> Fcn T_out/1
  W/1 -> Mux/2
  T_in/1 -> Mux/1

== system TruckBenchmark/Vehicle Model/ICE/Cylinder/lambda ==
  note: Avoid division by Zero
  W_ei : Inport
  W_f : Inport  Port=2
  X_Oim : Inport  Port=3
  Constant1 : Constant  Value=AFs*X_Oc
  Constant2 : Constant  Value=0
  Fcn : Fcn  Expr=(u[1]*u[3]-u[2]*AFs*X_Oc)/(u[1]+u[2])
  Fuel Limit : Constant  Value=1e-5
  Max1 : MinMax  Function=max  Inputs=2  InputSameDT=on  SaturateOnIntegerOverflow=on
  MinMax : MinMax  Function=max  Inputs=2  InputSameDT=on  SaturateOnIntegerOverflow=on
  Mux : Mux  Inputs=3
  lambda : Product  Inputs=/*/*  SaturateOnIntegerOverflow=on  OutDataTypeStr=Inherit: Same as first input
  lambda_out : Outport  VectorParamsAs1DForOutWhenUnconnected=off
  X_Oe : Outport  Port=2  VectorParamsAs1DForOutWhenUnconnected=off
  tag scope: lambda=global
  wires:
  Constant2/1 -> MinMax/2
  Fcn/1 -> MinMax/1
  MinMax/1 -> X_Oe/1
  Mux/1 -> Fcn/1
  X_Oim/1 -> Mux/3, lambda/4
  Max1/1 -> Mux/2, lambda/3
  W_ei/1 -> Mux/1, lambda/2
  lambda/1 -> lambda_out/1, [lambda]  "r_lambdaOut"
  Constant1/1 -> lambda/1
  Fuel Limit/1 -> Max1/2
  W_f/1 -> Max1/1

== system TruckBenchmark/Vehicle Model/ICE/EGR-system/EGR act ==
  In : Inport
  Actuator1 : Subsystem  mask{tau=model.engine.tau_egr1, uInit=model.engine.uInit_egr}
  Actuator2 : Subsystem  mask{tau=model.engine.tau_egr2, uInit=model.engine.uInit_egr}
  Gain : Gain  Gain=model.engine.K_egr
  Gain1 : Gain  Gain=model.engine.K_egr-1
  Subtract : Sum  Inputs=+-
  Transport Delay : TransportDelay  DelayTime=model.engine.tau_degr  InitialOutput=model.engine.uInit_egr
  Out : Outport  VectorParamsAs1DForOutWhenUnconnected=off
  wires:
  Gain1/1 -> Subtract/2
  Gain/1 -> Subtract/1
  Actuator2/1(Out) -> Gain1/1
  Actuator1/1(Out) -> Gain/1
  Transport Delay/1 -> Actuator2/1(In), Actuator1/1(In)
  Subtract/1 -> Out/1
  In/1 -> Transport Delay/1

== system TruckBenchmark/Vehicle Model/ICE/EGR-system/PSI_egr ==
  PI_egr : Inport
  PSI_egr function : Fcn  Expr=1-((1-u)/(1-PI_egropt)-1)^2
  Saturation : Saturate  UpperLimit=1  LowerLimit=PI_egropt
  PSI_egr : Outport  VectorParamsAs1DForOutWhenUnconnected=off
  wires:
  PSI_egr function/1 -> PSI_egr/1
  PI_egr/1 -> Saturation/1
  Saturation/1 -> PSI_egr function/1

== system TruckBenchmark/Vehicle Model/ICE/EGR-system/f_egr ==
  u_egr : Inport
  Constant : Constant  Value=0
  Constant1 : Constant  Value=-c_egr(2)/2/c_egr(1)
  MinMax : MinMax  Function=max  Inputs=2  InputSameDT=on  SaturateOnIntegerOverflow=on
  MinMax1 : MinMax  Inputs=2  InputSameDT=on  SaturateOnIntegerOverflow=on
  Polynomial : Polyval  Coefs=c_egr
  f_egr : Outport  VectorParamsAs1DForOutWhenUnconnected=off
  wires:
  Constant1/1 -> MinMax1/2
  MinMax1/1 -> Polynomial/1
  u_egr/1 -> MinMax1/1
  MinMax/1 -> f_egr/1
  Constant/1 -> MinMax/2
  Polynomial/1 -> MinMax/1

== system TruckBenchmark/Vehicle Model/ICE/Exhaust Manifold/Subsystem ==
  p_em : Inport
  T_em : Inport  Port=2
  W_eo : Inport  Port=3
  X_Oe : Inport  Port=4
  Fcn1 : Fcn  Expr=R_e*u[2]/u[1]/V_em*u[3]*(u[4]-u[5])
  Integrator X_Oem : Integrator  LimitOutput=on  UpperSaturationLimit=1  LowerSaturationLimit=0
  Mux1 : Mux  Inputs=5
  X_Oem : Outport  VectorParamsAs1DForOutWhenUnconnected=off
  wires:
  T_em/1 -> Mux1/2
  X_Oe/1 -> Mux1/4
  Integrator X_Oem/1 -> Mux1/5, X_Oem/1
  W_eo/1 -> Mux1/3
  p_em/1 -> Mux1/1
  Fcn1/1 -> Integrator X_Oem/1
  Mux1/1 -> Fcn1/1

== system TruckBenchmark/Vehicle Model/ICE/Intake Manifold/Subsystem X_Oim ==
  p_im : Inport
  T_im : Inport  Port=2
  W_egr : Inport  Port=3
  W_c : Inport  Port=4
  X_Oem : Inport  Port=5
  Fcn1 : Fcn  Expr=R_a*u[2]/u[1]/V_im*(u[3]*(u[5]-u[6])+u[4]*(X_Oc-u[6]))
  Integrator X_Oim : Integrator  InitialCondition=0.2314  LimitOutput=on  UpperSaturationLimit=1  LowerSaturationLimit=0
  Mux1 : Mux  Inputs=6
  X_Oim : Outport  VectorParamsAs1DForOutWhenUnconnected=off
  wires:
  X_Oem/1 -> Mux1/5
  Integrator X_Oim/1 -> Mux1/6, X_Oim/1
  W_c/1 -> Mux1/4
  W_egr/1 -> Mux1/3
  T_im/1 -> Mux1/2
  p_im/1 -> Mux1/1
  Mux1/1 -> Fcn1/1
  Fcn1/1 -> Integrator X_Oim/1

== system TruckBenchmark/Vehicle Model/ICE/Turbo/Compressor ==
  T_bc : Inport
  p_bc : Inport  Port=2
  p_c : Inport  Port=3
  omega_t : Inport  Port=4
  DeltaT_c : Subsystem
  Fcn P_c : Fcn  Expr=u[2]*c_pa*u[1]
  Mux1 : Mux  Inputs=2
  Sub PI_c : Subsystem
  Sub W_c : Subsystem
  Sum : Sum  SaturateOnIntegerOverflow=on
  W_c : Outport  VectorParamsAs1DForOutWhenUnconnected=off
  T_c : Outport  Port=2  VectorParamsAs1DForOutWhenUnconnected=off
  P_c : Outport  Port=3  VectorParamsAs1DForOutWhenUnconnected=off
  tag scope: P_c=global, W_c=global
  wires:
  Sum/1 -> T_c/1
  Fcn P_c/1 -> [P_c], P_c/1
  Sub W_c/1(W_c) -> W_c/1, [W_c], DeltaT_c/3(W_c), Mux1/2
  omega_t/1 -> Sub W_c/3(omega_t)
  T_bc/1 -> Sub W_c/2(T_bc), DeltaT_c/2(T_bc), Sum/2
  Mux1/1 -> Fcn P_c/1
  DeltaT_c/1(DeltaT_c) -> Sum/1, Mux1/1
  Sub PI_c/1(PI_c) -> DeltaT_c/1(PI_c), Sub W_c/1(PI_c)
  p_bc/1 -> Sub PI_c/2(p_bc), Sub W_c/4(p_bc)
  p_c/1 -> Sub PI_c/1(p_c)

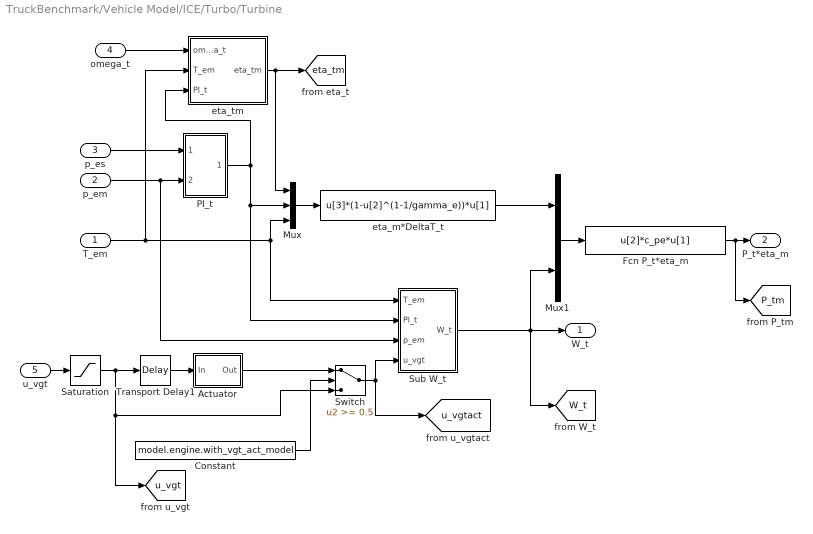
== system TruckBenchmark/Vehicle Model/ICE/Turbo/Turbine ==
  T_em : Inport
  p_em : Inport  Port=2
  p_es : Inport  Port=3
  omega_t : Inport  Port=4
  u_vgt : Inport  Port=5
  Actuator : Subsystem  mask{tau=tau_vgt, uInit=uInit_vgt}
  Constant : Constant  Value=model.engine.with_vgt_act_model
  Fcn P_t*eta_m : Fcn  Expr=u[2]*c_pe*u[1]
  Mux : Mux  Inputs=3
  Mux1 : Mux  Inputs=2
  PI_t : Subsystem
  Saturation : Saturate  UpperLimit=100  LowerLimit=20
  Sub W_t : Subsystem
  Switch : Switch  Threshold=0.5  InputSameDT=off
  Transport Delay1 : TransportDelay  DelayTime=model.engine.tau_dvgt  InitialOutput=model.engine.uInit_vgt
  eta_m*DeltaT_t : Fcn  Expr=u[3]*(1-u[2]^(1-1/gamma_e))*u[1]
  eta_tm : Subsystem
  W_t : Outport  VectorParamsAs1DForOutWhenUnconnected=off
  P_t*eta_m : Outport  Port=2  VectorParamsAs1DForOutWhenUnconnected=off
  tag scope: P_tm=global, W_t=global, eta_tm=global, u_vgt=global, u_vgtact=global
  wires:
  Switch/1 -> [u_vgtact], Sub W_t/4(u_vgt)
  Actuator/1(Out) -> Switch/1
  Constant/1 -> Switch/2
  Transport Delay1/1 -> Actuator/1(In)
  u_vgt/1 -> Saturation/1
  eta_tm/1(eta_tm) -> [eta_tm], Mux/1
  Sub W_t/1(W_t) -> [W_t], Mux1/2, W_t/1
  p_es/1 -> PI_t/1(p_es)
  p_em/1 -> Sub W_t/3(p_em), PI_t/2(p_em)
  PI_t/1(PI_t) -> eta_tm/3(PI_t), Sub W_t/2(PI_t), Mux/2
  Mux/1 -> eta_m*DeltaT_t/1
  eta_m*DeltaT_t/1 -> Mux1/1
  Mux1/1 -> Fcn P_t*eta_m/1
  T_em/1 -> eta_tm/2(T_em), Mux/3, Sub W_t/1(T_em)
  omega_t/1 -> eta_tm/1(omega_t)
  Fcn P_t*eta_m/1 -> [P_tm], P_t*eta_m/1
  Saturation/1 -> Switch/3, [u_vgt], Transport Delay1/1

== system TruckBenchmark/Vehicle Model/ICE/Turbo/Turbo inertia ==
  P_t*eta_m : Inport
  P_c : Inport  Port=2
  Divide : Product  Inputs=*/
  Gain : Gain  Gain=1/J_t  SaturateOnIntegerOverflow=on  OutDataTypeStr=Inherit: Same as input  ParamDataTypeStr=Inherit: Same as input
  Gain2 : Gain  Gain=30/pi  SaturateOnIntegerOverflow=on  OutDataTypeStr=Inherit: Same as input  ParamDataTypeStr=Inherit: Same as input
  Integrator omega_t : Integrator  InitialCondition=omega_t_Init  LimitOutput=on  UpperSaturationLimit=200000*pi/30  LowerSaturationLimit=100*pi/30
  Sum : Sum  Inputs=+-  SaturateOnIntegerOverflow=on
  omega_t : Outport  VectorParamsAs1DForOutWhenUnconnected=off
  tag scope: n_t=global
  wires:
  Integrator omega_t/1 -> omega_t/1, Gain2/1, Divide/2
  P_c/1 -> Sum/2
  P_t*eta_m/1 -> Sum/1
  Gain2/1 -> [n_t]
  Gain/1 -> Integrator omega_t/1
  Sum/1 -> Divide/1
  Divide/1 -> Gain/1

== system TruckBenchmark/Controller/CAN TX//RX/Attack Block/C-GAttack Block/If Action Subsystem ==
  Action Port : ActionPort  PropagateVarSize=During execution  ActionPortLabel=if(u1 <= 30)
  1-D Lookup Table : Lookup_n-D  NumberOfTableDimensions=1  BreakpointsForDimension1=ts.gen_30kph.Time  Table=ts.gen_30kph.Data  InternalRulePriority=Speed  RndMeth=Simplest
  Clock : Clock
  AttachSpd_30 : Outport
  wires:
  Clock/1 -> 1-D Lookup Table/1
  1-D Lookup Table/1 -> AttachSpd_30/1

== system TruckBenchmark/Controller/CAN TX//RX/Attack Block/C-GAttack Block/If Action Subsystem1 ==
  Action Port : ActionPort  PropagateVarSize=During execution  ActionPortLabel=elseif(u1 >= 31 & u1<=40)
  1-D Lookup Table : Lookup_n-D  NumberOfTableDimensions=1  BreakpointsForDimension1=ts.gen_40kph.Time  Table=ts.gen_40kph.Data  InternalRulePriority=Speed  RndMeth=Simplest
  Clock : Clock
  AttachSpd_40 : Outport
  wires:
  Clock/1 -> 1-D Lookup Table/1
  1-D Lookup Table/1 -> AttachSpd_40/1

== system TruckBenchmark/Controller/CAN TX//RX/Attack Block/C-GAttack Block/If Action Subsystem2 ==
  Action Port : ActionPort  PropagateVarSize=During execution  ActionPortLabel=elseif(u1 >= 41 & u1<=50)
  1-D Lookup Table : Lookup_n-D  NumberOfTableDimensions=1  BreakpointsForDimension1=ts.gen_50kph.Time  Table=ts.gen_50kph.Data  InternalRulePriority=Speed  RndMeth=Simplest
  Clock : Clock
  AttachSpd_50 : Outport
  wires:
  Clock/1 -> 1-D Lookup Table/1
  1-D Lookup Table/1 -> AttachSpd_50/1

== system TruckBenchmark/Controller/CAN TX//RX/Attack Block/C-GAttack Block/If Action Subsystem3 ==
  Action Port : ActionPort  PropagateVarSize=During execution  ActionPortLabel=elseif(u1 >= 51 & u1<=60)
  1-D Lookup Table : Lookup_n-D  NumberOfTableDimensions=1  BreakpointsForDimension1=ts.gen_60kph.Time  Table=ts.gen_60kph.Data  InternalRulePriority=Speed  RndMeth=Simplest
  Clock : Clock
  AttachSpd_60 : Outport
  wires:
  Clock/1 -> 1-D Lookup Table/1
  1-D Lookup Table/1 -> AttachSpd_60/1

== system TruckBenchmark/Controller/CAN TX//RX/Attack Block/C-GAttack Block/If Action Subsystem4 ==
  Action Port : ActionPort  PropagateVarSize=During execution  ActionPortLabel=elseif(u1 >= 61 & u1<=70)
  1-D Lookup Table : Lookup_n-D  NumberOfTableDimensions=1  BreakpointsForDimension1=ts.gen_70kph.Time  Table=ts.gen_70kph.Data  InternalRulePriority=Speed  RndMeth=Simplest
  Clock : Clock
  AttachSpd_70 : Outport
  wires:
  Clock/1 -> 1-D Lookup Table/1
  1-D Lookup Table/1 -> AttachSpd_70/1

== system TruckBenchmark/Controller/CAN TX//RX/Attack Block/C-GAttack Block/If Action Subsystem5 ==
  Action Port : ActionPort  PropagateVarSize=During execution  ActionPortLabel=elseif(u1 >= 81 & u1<=90)
  1-D Lookup Table : Lookup_n-D  NumberOfTableDimensions=1  BreakpointsForDimension1=ts.gen_90kph.Time  Table=ts.gen_90kph.Data  InternalRulePriority=Speed  RndMeth=Simplest
  Clock : Clock
  AttackSpd_90 : Outport
  wires:
  Clock/1 -> 1-D Lookup Table/1
  1-D Lookup Table/1 -> AttackSpd_90/1

== system TruckBenchmark/Controller/CAN TX//RX/Attack Block/C-GAttack Block/If Action Subsystem6 ==
  Action Port : ActionPort  PropagateVarSize=During execution  ActionPortLabel=elseif(u1 >= 71 & u1<=80)
  1-D Lookup Table : Lookup_n-D  NumberOfTableDimensions=1  BreakpointsForDimension1=ts.gen_80kph.Time  Table=ts.gen_80kph.Data  InternalRulePriority=Speed  RndMeth=Simplest
  Clock : Clock
  AttachSpd_80 : Outport
  wires:
  Clock/1 -> 1-D Lookup Table/1
  1-D Lookup Table/1 -> AttachSpd_80/1

== system TruckBenchmark/Vehicle Model/ICE/Cylinder/Cylinder temp (one iter with delay)/Sub T_e ==
  PI_e : Inport
  q_in : Inport  Port=2
  T1 : Inport  Port=3
  x_p : Inport  Port=4
  Fcn T_e : Fcn  Expr=eta_sc*u[1]^(1-1/gamma_a)*r_c^(1-gamma_a)*u[4]^(1/gamma_a-1)*(u[2]*((1-x_cv)/c_pa+x_cv/c_va)+u[3]*r_c^(gamma_a-1))
  Mux2 : Mux
  T_e : Outport  VectorParamsAs1DForOutWhenUnconnected=off
  wires:
  Fcn T_e/1 -> T_e/1
  x_p/1 -> Mux2/4
  T1/1 -> Mux2/3
  q_in/1 -> Mux2/2
  PI_e/1 -> Mux2/1
  Mux2/1 -> Fcn T_e/1

== system TruckBenchmark/Vehicle Model/ICE/Cylinder/Cylinder temp (one iter with delay)/x_p ==
  q_in : Inport
  T1 : Inport  Port=2
  Fcn x_p : Fcn  Expr=1+u[1]*x_cv/(c_va*u[2]*r_c^(gamma_a-1))
  Mux1 : Mux  Inputs=2
  x_p : Outport  VectorParamsAs1DForOutWhenUnconnected=off
  wires:
  Fcn x_p/1 -> x_p/1
  T1/1 -> Mux1/2
  q_in/1 -> Mux1/1
  Mux1/1 -> Fcn x_p/1

== system TruckBenchmark/Vehicle Model/ICE/Cylinder/Cylinder temp (one iter with delay)/x_r ==
  x_p : Inport
  T1 : Inport  Port=2
  q_in : Inport  Port=3
  PI_e : Inport  Port=4
  Fcn x_r : Fcn  Expr=u[3]^(1/gamma_a)*u[1]^(-1/gamma_a)/(r_c*u[2])
  Mux4 : Mux  Inputs=2
  Mux5 : Mux  Inputs=3
  x_v : Fcn  Expr=1+u[2]*(1-x_cv)/(c_pa*(u[2]*x_cv/c_va+u[1]*r_c^(gamma_a-1)))
  x_r : Outport  VectorParamsAs1DForOutWhenUnconnected=off
  wires:
  PI_e/1 -> Mux5/3
  q_in/1 -> Mux4/2
  T1/1 -> Mux4/1
  x_p/1 -> Mux5/1
  x_v/1 -> Mux5/2
  Fcn x_r/1 -> x_r/1
  Mux5/1 -> Fcn x_r/1
  Mux4/1 -> x_v/1

== system TruckBenchmark/Vehicle Model/ICE/EGR-system/EGR act/Actuator1 ==
  In : Inport
  Gain : Gain  Gain=1/tau  SaturateOnIntegerOverflow=on  OutDataTypeStr=Inherit: Same as input  ParamDataTypeStr=Inherit: Same as input
  Integrator : Integrator  InitialCondition=uInit
  Sum : Sum  Inputs=|+-  SaturateOnIntegerOverflow=on
  Out : Outport  VectorParamsAs1DForOutWhenUnconnected=off
  wires:
  Gain/1 -> Integrator/1
  Sum/1 -> Gain/1
  Integrator/1 -> Out/1, Sum/2
  In/1 -> Sum/1

== system TruckBenchmark/Vehicle Model/ICE/EGR-system/EGR act/Actuator2 ==
  In : Inport
  Gain : Gain  Gain=1/tau  SaturateOnIntegerOverflow=on  OutDataTypeStr=Inherit: Same as input  ParamDataTypeStr=Inherit: Same as input
  Integrator : Integrator  InitialCondition=uInit
  Sum : Sum  Inputs=|+-  SaturateOnIntegerOverflow=on
  Out : Outport  VectorParamsAs1DForOutWhenUnconnected=off
  wires:
  Gain/1 -> Integrator/1
  Sum/1 -> Gain/1
  Integrator/1 -> Out/1, Sum/2
  In/1 -> Sum/1

== system TruckBenchmark/Vehicle Model/ICE/Turbo/Compressor/DeltaT_c ==
  PI_c : Inport
  T_bc : Inport  Port=2
  W_c : Inport  Port=3
  Fcn DeltaT_c : Fcn  Expr=u[3]*(u[2]^(1-1/gamma_a)-1)/u[1]
  Mux : Mux  Inputs=3
  eta_c : Subsystem
  DeltaT_c : Outport  VectorParamsAs1DForOutWhenUnconnected=off
  tag scope: eta_c=global
  wires:
  Fcn DeltaT_c/1 -> DeltaT_c/1
  T_bc/1 -> Mux/3
  PI_c/1 -> Mux/2, eta_c/2(PI_c)
  W_c/1 -> eta_c/1(W_c)
  eta_c/1(eta_c) -> [eta_c], Mux/1
  Mux/1 -> Fcn DeltaT_c/1

== system TruckBenchmark/Vehicle Model/ICE/Turbo/Compressor/Sub PI_c ==
  p_c : Inport
  p_bc : Inport  Port=2
  Constant1 : Constant
  Div PI_c : Product  Inputs=*/  SaturateOnIntegerOverflow=on  OutDataTypeStr=Inherit: Same as first input
  MinMax1 : MinMax  Function=max  Inputs=2  InputSameDT=on  SaturateOnIntegerOverflow=on
  PI_c : Outport  VectorParamsAs1DForOutWhenUnconnected=off
  wires:
  MinMax1/1 -> PI_c/1
  p_c/1 -> Div PI_c/1
  p_bc/1 -> Div PI_c/2
  Constant1/1 -> MinMax1/2
  Div PI_c/1 -> MinMax1/1

== system TruckBenchmark/Vehicle Model/ICE/Turbo/Compressor/Sub W_c ==
  PI_c : Inport
  T_bc : Inport  Port=2
  omega_t : Inport  Port=3
  p_bc : Inport  Port=4
  Fcn W_c : Fcn  Expr=u[3]*pi*R_c^3*u[1]*u[4]/(R_a*u[2])
  Mux3 : Mux
  PHI_c : Subsystem
  Saturation : Saturate  UpperLimit=inf  LowerLimit=1e-4
  W_c : Outport  VectorParamsAs1DForOutWhenUnconnected=off
  wires:
  Saturation/1 -> W_c/1  "dm_airInlet"
  Fcn W_c/1 -> Saturation/1
  PI_c/1 -> PHI_c/1(PI_c)
  p_bc/1 -> Mux3/3
  T_bc/1 -> Mux3/2, PHI_c/2(T_bc)
  omega_t/1 -> Mux3/1, PHI_c/3(omega_t)
  PHI_c/1(PHI_c) -> Mux3/4
  Mux3/1 -> Fcn W_c/1

== system TruckBenchmark/Vehicle Model/ICE/Turbo/Turbine/Actuator ==
  In : Inport
  Gain : Gain  Gain=1/tau  SaturateOnIntegerOverflow=on  OutDataTypeStr=Inherit: Same as input  ParamDataTypeStr=Inherit: Same as input
  Integrator : Integrator  InitialCondition=uInit
  Sum : Sum  Inputs=|+-  SaturateOnIntegerOverflow=on
  Out : Outport  VectorParamsAs1DForOutWhenUnconnected=off
  wires:
  Gain/1 -> Integrator/1
  Sum/1 -> Gain/1
  Integrator/1 -> Out/1, Sum/2
  In/1 -> Sum/1

== system TruckBenchmark/Vehicle Model/ICE/Turbo/Turbine/PI_t ==
  p_es : Inport
  p_em : Inport  Port=2
  Constant : Constant  Value=0.9999
  Div PI_t : Product  Inputs=*/  SaturateOnIntegerOverflow=on  OutDataTypeStr=Inherit: Same as first input
  MinMax : MinMax  Inputs=2  InputSameDT=on  SaturateOnIntegerOverflow=on
  PI_t : Outport  VectorParamsAs1DForOutWhenUnconnected=off
  wires:
  MinMax/1 -> PI_t/1
  p_es/1 -> Div PI_t/1
  p_em/1 -> Div PI_t/2
  Div PI_t/1 -> MinMax/1
  Constant/1 -> MinMax/2

== system TruckBenchmark/Vehicle Model/ICE/Turbo/Turbine/Sub W_t ==
  T_em : Inport
  PI_t : Inport  Port=2
  p_em : Inport  Port=3
  u_vgt : Inport  Port=4
  Fcn W_t : Fcn  Expr=A_vgtmax*u[3]*sqrt(1-u[2]^K_t)*u[4]/sqrt(u[1]*R_e)
  Mux3 : Mux
  f_vgt : Subsystem
  W_t : Outport  VectorParamsAs1DForOutWhenUnconnected=off
  wires:
  u_vgt/1 -> f_vgt/1(u_vgt)
  Fcn W_t/1 -> W_t/1
  p_em/1 -> Mux3/3
  PI_t/1 -> Mux3/2
  T_em/1 -> Mux3/1
  f_vgt/1(f_vgt) -> Mux3/4
  Mux3/1 -> Fcn W_t/1
